simulink model "BBC_ensemble_other"  (R2022a)
settings: Solver=ode15s  StartTime=0.0  StopTime=Tf  RelTol=1e-3  AbsTol=1e-3
PreLoadFcn:
  | Jdamping = 1e-4;
values from neighbouring files (symbols this model uses):
  ball = evalin('base','ball')    [animatedPath.m]
  g = 9.80665    [kinova_params.m]
  max_torque = 0.25    [kinova_params.m]
  plate = evalin('base','plate')    [animatedPath.m]
  R1_q0 = 0    [kinova_params.m]
  R2_q0 = deg2rad(20)    [kinova_params.m]
  R3_q0 = 0    [kinova_params.m]
  R4_q0 = deg2rad(135)    [kinova_params.m]
  R5_q0 = 0    [kinova_params.m]
  U0 = [wrist_torque_0 hand_torque_0]    [kinova_params.m]
undefined symbols (not defined in the file or in its folder): actionTable, actionToIndex, actionUB1, actionUB2, ballWeight, isAvg, isPred, isTerminate, isVote, plateWeight, rewardToIndex, rewardUB1, rewardUB2, stableWeight, stateTable, tranTable, X, Y, Z
libraries: sm_lib x96, nesl_utility x18, rllib x9, dspstat3 x2, simulink x2
(part 3 of 3)

== system BBC_ensemble_other/Kinova Ball Balance/7 DOF Manipulator/Wrist1_Link ==
  Actuator5_AxisInvTransform : sm_lib/Frames and Transforms/Rigid Transform  TranslationMethod=Cartesian  TranslationStandardOffset=0  TranslationLengthUnit=m  TranslationStandardAxis=+Z  TranslationCartesianOffset=[0, 0, 0]  TranslationROffset=0  TranslationROffsetUnits=m  TranslationZOffset=0  TranslationZOffsetUnits=m  TranslationThetaOffset=0  TranslationThetaOffsetUnits=deg  RotationMethod=ArbitraryAxis  RotationAngleUnits=rad  RotationStandardAxis=+Z  RotationAngle=0  RotationArbitraryAxis=[1, 0, 0]  FollAlignAxisA=+X  BaseAlignAxisA=+Y  FollAlignAxisB=+Y  BaseAlignAxisB=+Z  RotationSequenceAxes=FollowerAxes  RotationSequence=XYX  RotationSequenceAngles=[0 0 0]  RotationSequenceAnglesUnits=deg  RotationMatrix=[1 0 0; 0 1 0; 0 0 1]
  Actuator6_AxisTransform : sm_lib/Frames and Transforms/Rigid Transform  TranslationMethod=Cartesian  TranslationStandardOffset=0  TranslationLengthUnit=m  TranslationStandardAxis=+Z  TranslationCartesianOffset=[0, 0, 0]  TranslationROffset=0  TranslationROffsetUnits=m  TranslationZOffset=0  TranslationZOffsetUnits=m  TranslationThetaOffset=0  TranslationThetaOffsetUnits=deg  RotationMethod=ArbitraryAxis  RotationAngleUnits=rad  RotationStandardAxis=+Z  RotationAngle=0  RotationArbitraryAxis=[1, 0, 0]  FollAlignAxisA=+X  BaseAlignAxisA=+Y  FollAlignAxisB=+Y  BaseAlignAxisB=+Z  RotationSequenceAxes=FollowerAxes  RotationSequence=XYX  RotationSequenceAngles=[0 0 0]  RotationSequenceAnglesUnits=deg  RotationMatrix=[1 0 0; 0 1 0; 0 0 1]
  Actuator6_OriginTransform : sm_lib/Frames and Transforms/Rigid Transform  TranslationMethod=Cartesian  TranslationStandardOffset=0  TranslationLengthUnit=m  TranslationStandardAxis=+Z  TranslationCartesianOffset=[0, 0.00017505, -0.10593]  TranslationROffset=0  TranslationROffsetUnits=m  TranslationZOffset=0  TranslationZOffsetUnits=m  TranslationThetaOffset=0  TranslationThetaOffsetUnits=deg  RotationMethod=RotationSequence  RotationAngleUnits=deg  RotationStandardAxis=+Z  RotationAngle=0.0  RotationArbitraryAxis=[0 0 1]  FollAlignAxisA=+X  BaseAlignAxisA=+Y  FollAlignAxisB=+Y  BaseAlignAxisB=+Z  RotationSequenceAxes=BaseAxes  RotationSequence=XYZ  RotationSequenceAngles=[1.5708, 0, 0]  RotationSequenceAnglesUnits=rad  RotationMatrix=[1 0 0; 0 1 0; 0 0 1]
  Inertia : sm_lib/Body Elements/Inertia  InertiaType=Custom  Mass=0.654  MassUnits=kg  CenterOfMass=[0, 0, 0]  CenterOfMassUnits=m  MomentsOfInertia=[0.0013311, 0.0013282, 0.00030696]  MomentsOfInertiaUnits=kg*m^2  ProductsOfInertia=[-0.00022936, -4.267800000000005e-10, -4.584900000000001e-10]  ProductsOfInertiaUnits=kg*m^2  GraphicType=None  MarkerShape=Inertia  MarkerSize=20  GraphicVisPropType=SimpleVisualProperties  GraphicDiffuseColor=[0.5 0.5 0.5]  GraphicSpecularColor=[0.5 0.5 0.5 1.0]  GraphicAmbientColor=[0.15 0.15 0.15 1.0]  GraphicEmissiveColor=[0.0 0.0 0.0 1.0]  GraphicShininess=75  GraphicOpacity=1.0
  InertiaOriginTransform : sm_lib/Frames and Transforms/Rigid Transform  TranslationMethod=Cartesian  TranslationStandardOffset=0  TranslationLengthUnit=m  TranslationStandardAxis=+Z  TranslationCartesianOffset=[-3.2964e-07, -0.009617000000000001, -0.062968]  TranslationROffset=0  TranslationROffsetUnits=m  TranslationZOffset=0  TranslationZOffsetUnits=m  TranslationThetaOffset=0  TranslationThetaOffsetUnits=deg  RotationMethod=RotationSequence  RotationAngleUnits=deg  RotationStandardAxis=+Z  RotationAngle=0.0  RotationArbitraryAxis=[0 0 1]  FollAlignAxisA=+X  BaseAlignAxisA=+Y  FollAlignAxisB=+Y  BaseAlignAxisB=+Z  RotationSequenceAxes=BaseAxes  RotationSequence=XYZ  RotationSequenceAngles=[0, 0, 0]  RotationSequenceAnglesUnits=rad  RotationMatrix=[1 0 0; 0 1 0; 0 0 1]
  ReferenceFrame : sm_lib/Frames and Transforms/Reference Frame
  VisualOriginTransform : sm_lib/Frames and Transforms/Rigid Transform  TranslationMethod=Cartesian  TranslationStandardOffset=0  TranslationLengthUnit=m  TranslationStandardAxis=+Z  TranslationCartesianOffset=[0, 0, 0]  TranslationROffset=0  TranslationROffsetUnits=m  TranslationZOffset=0  TranslationZOffsetUnits=m  TranslationThetaOffset=0  TranslationThetaOffsetUnits=deg  RotationMethod=RotationSequence  RotationAngleUnits=deg  RotationStandardAxis=+Z  RotationAngle=0.0  RotationArbitraryAxis=[0 0 1]  FollAlignAxisA=+X  BaseAlignAxisA=+Y  FollAlignAxisB=+Y  BaseAlignAxisB=+Z  RotationSequenceAxes=BaseAxes  RotationSequence=XYZ  RotationSequenceAngles=[0, 0, 0]  RotationSequenceAnglesUnits=rad  RotationMatrix=[1 0 0; 0 1 0; 0 0 1]
  Wrist1 Link : Subsystem  Variant=on  VariantControlMode=label  VariantControl=Choice  LabelModeActiveChoice=Choice
  F : PMIOPort  Side=Left
  F1 : PMIOPort  Port=2  Side=Right
  connections:
  Actuator5_AxisInvTransform/RConn1 -- F/RConn1
  Actuator6_AxisTransform/RConn1 -- F1/RConn1
  Actuator6_AxisTransform/LConn1 -- Actuator6_OriginTransform/RConn1
  Inertia/RConn1 -- InertiaOriginTransform/RConn1
  Actuator6_OriginTransform/LConn1 -- Actuator5_AxisInvTransform/LConn1 -- InertiaOriginTransform/LConn1 -- VisualOriginTransform/LConn1 -- ReferenceFrame/RConn1
  VisualOriginTransform/RConn1 -- Wrist1 Link/RConn1

== system BBC_ensemble_other/Kinova Ball Balance/7 DOF Manipulator/Wrist2_Link ==
  Actuator6_AxisInvTransform : sm_lib/Frames and Transforms/Rigid Transform  TranslationMethod=Cartesian  TranslationStandardOffset=0  TranslationLengthUnit=m  TranslationStandardAxis=+Z  TranslationCartesianOffset=[0, 0, 0]  TranslationROffset=0  TranslationROffsetUnits=m  TranslationZOffset=0  TranslationZOffsetUnits=m  TranslationThetaOffset=0  TranslationThetaOffsetUnits=deg  RotationMethod=ArbitraryAxis  RotationAngleUnits=rad  RotationStandardAxis=+Z  RotationAngle=0  RotationArbitraryAxis=[1, 0, 0]  FollAlignAxisA=+X  BaseAlignAxisA=+Y  FollAlignAxisB=+Y  BaseAlignAxisB=+Z  RotationSequenceAxes=FollowerAxes  RotationSequence=XYX  RotationSequenceAngles=[0 0 0]  RotationSequenceAnglesUnits=deg  RotationMatrix=[1 0 0; 0 1 0; 0 0 1]
  Actuator7_AxisTransform : sm_lib/Frames and Transforms/Rigid Transform  TranslationMethod=Cartesian  TranslationStandardOffset=0  TranslationLengthUnit=m  TranslationStandardAxis=+Z  TranslationCartesianOffset=[0, 0, 0]  TranslationROffset=0  TranslationROffsetUnits=m  TranslationZOffset=0  TranslationZOffsetUnits=m  TranslationThetaOffset=0  TranslationThetaOffsetUnits=deg  RotationMethod=ArbitraryAxis  RotationAngleUnits=rad  RotationStandardAxis=+Z  RotationAngle=0  RotationArbitraryAxis=[1, 0, 0]  FollAlignAxisA=+X  BaseAlignAxisA=+Y  FollAlignAxisB=+Y  BaseAlignAxisB=+Z  RotationSequenceAxes=FollowerAxes  RotationSequence=XYX  RotationSequenceAngles=[0 0 0]  RotationSequenceAnglesUnits=deg  RotationMatrix=[1 0 0; 0 1 0; 0 0 1]
  Actuator7_OriginTransform : sm_lib/Frames and Transforms/Rigid Transform  TranslationMethod=Cartesian  TranslationStandardOffset=0  TranslationLengthUnit=m  TranslationStandardAxis=+Z  TranslationCartesianOffset=[0, -0.10593, -0.00017505]  TranslationROffset=0  TranslationROffsetUnits=m  TranslationZOffset=0  TranslationZOffsetUnits=m  TranslationThetaOffset=0  TranslationThetaOffsetUnits=deg  RotationMethod=RotationSequence  RotationAngleUnits=deg  RotationStandardAxis=+Z  RotationAngle=0.0  RotationArbitraryAxis=[0 0 1]  FollAlignAxisA=+X  BaseAlignAxisA=+Y  FollAlignAxisB=+Y  BaseAlignAxisB=+Z  RotationSequenceAxes=BaseAxes  RotationSequence=XYZ  RotationSequenceAngles=[-1.5708, 0, 0]  RotationSequenceAnglesUnits=rad  RotationMatrix=[1 0 0; 0 1 0; 0 0 1]
  Inertia : sm_lib/Body Elements/Inertia  InertiaType=Custom  Mass=0.654  MassUnits=kg  CenterOfMass=[0, 0, 0]  CenterOfMassUnits=m  MomentsOfInertia=[0.0013422, 0.00031025, 0.001336]  MomentsOfInertiaUnits=kg*m^2  ProductsOfInertia=[0.00023506, -7.338199999999999e-10, 4.959600000000004e-10]  ProductsOfInertiaUnits=kg*m^2  GraphicType=None  MarkerShape=Inertia  MarkerSize=20  GraphicVisPropType=SimpleVisualProperties  GraphicDiffuseColor=[0.5 0.5 0.5]  GraphicSpecularColor=[0.5 0.5 0.5 1.0]  GraphicAmbientColor=[0.15 0.15 0.15 1.0]  GraphicEmissiveColor=[0.0 0.0 0.0 1.0]  GraphicShininess=75  GraphicOpacity=1.0
  InertiaOriginTransform : sm_lib/Frames and Transforms/Rigid Transform  TranslationMethod=Cartesian  TranslationStandardOffset=0  TranslationLengthUnit=m  TranslationStandardAxis=+Z  TranslationCartesianOffset=[-3.4377e-07, -0.044043, -0.0097804]  TranslationROffset=0  TranslationROffsetUnits=m  TranslationZOffset=0  TranslationZOffsetUnits=m  TranslationThetaOffset=0  TranslationThetaOffsetUnits=deg  RotationMethod=RotationSequence  RotationAngleUnits=deg  RotationStandardAxis=+Z  RotationAngle=0.0  RotationArbitraryAxis=[0 0 1]  FollAlignAxisA=+X  BaseAlignAxisA=+Y  FollAlignAxisB=+Y  BaseAlignAxisB=+Z  RotationSequenceAxes=BaseAxes  RotationSequence=XYZ  RotationSequenceAngles=[0, 0, 0]  RotationSequenceAnglesUnits=rad  RotationMatrix=[1 0 0; 0 1 0; 0 0 1]
  ReferenceFrame : sm_lib/Frames and Transforms/Reference Frame
  VisualOriginTransform : sm_lib/Frames and Transforms/Rigid Transform  TranslationMethod=Cartesian  TranslationStandardOffset=0  TranslationLengthUnit=m  TranslationStandardAxis=+Z  TranslationCartesianOffset=[0, 0, 0]  TranslationROffset=0  TranslationROffsetUnits=m  TranslationZOffset=0  TranslationZOffsetUnits=m  TranslationThetaOffset=0  TranslationThetaOffsetUnits=deg  RotationMethod=RotationSequence  RotationAngleUnits=deg  RotationStandardAxis=+Z  RotationAngle=0.0  RotationArbitraryAxis=[0 0 1]  FollAlignAxisA=+X  BaseAlignAxisA=+Y  FollAlignAxisB=+Y  BaseAlignAxisB=+Z  RotationSequenceAxes=BaseAxes  RotationSequence=XYZ  RotationSequenceAngles=[0, 0, 0]  RotationSequenceAnglesUnits=rad  RotationMatrix=[1 0 0; 0 1 0; 0 0 1]
  Wrist2 Link : Subsystem  Variant=on  VariantControlMode=label  VariantControl=Choice  LabelModeActiveChoice=Choice
  F : PMIOPort  Side=Left
  F1 : PMIOPort  Port=2  Side=Right
  connections:
  Actuator6_AxisInvTransform/RConn1 -- F/RConn1
  Actuator7_AxisTransform/RConn1 -- F1/RConn1
  Actuator7_AxisTransform/LConn1 -- Actuator7_OriginTransform/RConn1
  Inertia/RConn1 -- InertiaOriginTransform/RConn1
  Actuator7_OriginTransform/LConn1 -- Actuator6_AxisInvTransform/LConn1 -- InertiaOriginTransform/LConn1 -- VisualOriginTransform/LConn1 -- ReferenceFrame/RConn1
  VisualOriginTransform/RConn1 -- Wrist2 Link/RConn1

== system BBC_ensemble_other/Kinova Ball Balance/7 DOF Manipulator/base_link ==
  Actuator1_AxisTransform : sm_lib/Frames and Transforms/Rigid Transform  TranslationMethod=Cartesian  TranslationStandardOffset=0  TranslationLengthUnit=m  TranslationStandardAxis=+Z  TranslationCartesianOffset=[0, 0, 0]  TranslationROffset=0  TranslationROffsetUnits=m  TranslationZOffset=0  TranslationZOffsetUnits=m  TranslationThetaOffset=0  TranslationThetaOffsetUnits=deg  RotationMethod=ArbitraryAxis  RotationAngleUnits=rad  RotationStandardAxis=+Z  RotationAngle=0  RotationArbitraryAxis=[1, 0, 0]  FollAlignAxisA=+X  BaseAlignAxisA=+Y  FollAlignAxisB=+Y  BaseAlignAxisB=+Z  RotationSequenceAxes=FollowerAxes  RotationSequence=XYX  RotationSequenceAngles=[0 0 0]  RotationSequenceAnglesUnits=deg  RotationMatrix=[1 0 0; 0 1 0; 0 0 1]
  Actuator1_OriginTransform : sm_lib/Frames and Transforms/Rigid Transform  TranslationMethod=Cartesian  TranslationStandardOffset=0  TranslationLengthUnit=m  TranslationStandardAxis=+Z  TranslationCartesianOffset=[0, 0, 0.15643]  TranslationROffset=0  TranslationROffsetUnits=m  TranslationZOffset=0  TranslationZOffsetUnits=m  TranslationThetaOffset=0  TranslationThetaOffsetUnits=deg  RotationMethod=RotationSequence  RotationAngleUnits=deg  RotationStandardAxis=+Z  RotationAngle=0.0  RotationArbitraryAxis=[0 0 1]  FollAlignAxisA=+X  BaseAlignAxisA=+Y  FollAlignAxisB=+Y  BaseAlignAxisB=+Z  RotationSequenceAxes=BaseAxes  RotationSequence=XYZ  RotationSequenceAngles=[-3.141585307179587, 0, 0]  RotationSequenceAnglesUnits=rad  RotationMatrix=[1 0 0; 0 1 0; 0 0 1]
  Base Link : Subsystem  Variant=on  VariantControlMode=label  VariantControl=Choice  LabelModeActiveChoice=Choice
  ReferenceFrame : sm_lib/Frames and Transforms/Reference Frame
  F : PMIOPort  Side=Left
  F1 : PMIOPort  Port=2  Side=Right
  connections:
  Actuator1_AxisTransform/RConn1 -- F1/RConn1
  Actuator1_AxisTransform/LConn1 -- Actuator1_OriginTransform/RConn1
  F/RConn1 -- Actuator1_OriginTransform/LConn1 -- ReferenceFrame/RConn1 -- Base Link/RConn1

== system BBC_ensemble_other/Kinova Ball Balance/7 DOF Manipulator/mount ==
  Cylindrical Solid : sm_lib/Body Elements/Cylindrical Solid  GraphicAmbientColor=[0.15 0.15 0.15 1.0]  BasedOnType=Density  CenterOfMass=[0 0 0]  CenterOfMassUnits=m  GraphicDiffuseColor=[0.6 0.6 0.6]  CylinderLength=0.01  CylinderLengthUnits=m  CylinderRadius=0.1  CylinderRadiusUnits=m  Density=1000  DensityUnits=kg/m^3  DoExposeReferenceFrame=off  GraphicEmissiveColor=[0.0 0.0 0.0 1.0]  ExportEntireGeometry=off  SerializedFrames=<Frames><Frame><Id>Frame1</Id><Value><Name>F1</Name><Origin><Source>GeometricFeature</Source><FeatureName>top surface</FeatureName></Origin><PrimaryAxis><DefinedDirection>+Z</DefinedDirection><Source>ReferenceFrame</Source><SourceDirection>+Z</SourceDirection><FeatureName></FeatureName></PrimaryAxis><SecondaryAxis><DefinedDirection>+X</DefinedDirection><Source>ReferenceFrame</Source><SourceDirection>+X</SourceDirection><FeatureName></FeatureName></SecondaryAxis></Value></Frame><Frame><Id>Frame2</Id><Value><Name>F2</Name><Origin><Source>GeometricFeature</Source><FeatureName>bottom surface</FeatureName></Origin><PrimaryAxis><DefinedDirection>+Z</DefinedDirection><Source>ReferenceFrame</Source><SourceDirection>+Z</SourceDirection><FeatureName></FeatureName></PrimaryAxis><SecondaryAxis><DefinedDirection>+X</DefinedDirection><Source>ReferenceFrame</Source><SourceDirection>+X</SourceDirection><FeatureName></FeatureName></SecondaryAxis></Value></Frame></Frames>  MarkerShape=Sphere  MarkerSize=10  GraphicType=FromGeometry  InertiaType=CalculateFromGeometry  Mass=1  MassUnits=kg  MomentsOfInertia=[1 1 1]  MomentsOfInertiaUnits=kg*m^2  GraphicOpacity=1.0  ProductsOfInertia=[0 0 0]  ProductsOfInertiaUnits=kg*m^2  GraphicShininess=75  GraphicSpecularColor=[0.5 0.5 0.5 1.0]  GraphicVisPropType=SimpleVisualProperties
  F : PMIOPort  Side=Right
  F1 : PMIOPort  Port=2  Side=Left
  connections:
  Cylindrical Solid/LConn1 -- F1/RConn1
  F/RConn1 -- Cylindrical Solid/RConn1

== system BBC_ensemble_other/Kinova Ball Balance/7 DOF Manipulator/Bracelet_Link/Bracelet Link ==
  FileSolid : Subsystem  VariantControl=Choice_1
  Inertia : Subsystem  VariantControl=Choice
  R : PMIOPort  Side=Right

== system BBC_ensemble_other/Kinova Ball Balance/7 DOF Manipulator/ForeArm_Link/ForeArm Link ==
  FileSolid : Subsystem  VariantControl=Choice_1
  Inertia : Subsystem  VariantControl=Choice
  R : PMIOPort  Side=Right

== system BBC_ensemble_other/Kinova Ball Balance/7 DOF Manipulator/HalfArm1_Link/HalfArm1 Link ==
  FileSolid : Subsystem  VariantControl=Choice_1
  Inertia : Subsystem  VariantControl=Choice
  R : PMIOPort  Side=Right

== system BBC_ensemble_other/Kinova Ball Balance/7 DOF Manipulator/HalfArm2_Link/HalfArm2 Link ==
  FileSolid : Subsystem  VariantControl=Choice_1
  Inertia : Subsystem  VariantControl=Choice
  R : PMIOPort  Side=Right

== system BBC_ensemble_other/Kinova Ball Balance/7 DOF Manipulator/Shoulder_Link/Shoulder Link ==
  FileSolid : Subsystem  VariantControl=Choice_1
  Inertia : Subsystem  VariantControl=Choice
  R : PMIOPort  Side=Right

== system BBC_ensemble_other/Kinova Ball Balance/7 DOF Manipulator/Wrist1_Link/Wrist1 Link ==
  FileSolid : Subsystem  VariantControl=Choice_1
  Inertia : Subsystem  VariantControl=Choice
  R : PMIOPort  Side=Right

== system BBC_ensemble_other/Kinova Ball Balance/7 DOF Manipulator/Wrist2_Link/Wrist2 Link ==
  FileSolid : Subsystem  VariantControl=Choice_1
  Inertia : Subsystem  VariantControl=Choice
  R : PMIOPort  Side=Right

== system BBC_ensemble_other/Kinova Ball Balance/7 DOF Manipulator/base_link/Base Link ==
  FileSolid : Subsystem  VariantControl=Choice_1
  Inertia : Subsystem  VariantControl=Choice
  R : PMIOPort  Side=Right

== system BBC_ensemble_other/Kinova Ball Balance/7 DOF Manipulator/Bracelet_Link/Bracelet Link/FileSolid ==
  Bracelet Link : sm_lib/Body Elements/File Solid  ExtGeomFileName=bracelet_with_vision_link.STL  UnitType=Custom  ExtGeomFileUnits=m  StepReaderType=HEX  ExportConvexHullGeometry=off  InertiaType=Custom  Mass=0.0639903  MassUnits=kg  CenterOfMass=[-0.000374733, 0.0200972, 0.0397002]  CenterOfMassUnits=m  MomentsOfInertia=[8.77763e-05, 5.386e-05, 0.000111032]  MomentsOfInertiaUnits=kg*m^2  ProductsOfInertia=[-7.81917e-06, 1.77829e-07, -4.01652e-07]  ProductsOfInertiaUnits=kg*m^2  BasedOnType=DensityFromFile  Density=1000  DensityUnits=kg/m^3  DoExposeReferenceFrame=on  SerializedFrames=<Frames/>  GraphicType=FromGeometry  MarkerShape=Sphere  MarkerSize=10  GraphicVisPropType=SimpleVisualProperties  GraphicDiffuseColor=[0.6666667 0.77254903 0.92941177]  GraphicSpecularColor=[0.5 0.5 0.5 1.0]  GraphicAmbientColor=[0.15 0.15 0.15 1.0]  GraphicEmissiveColor=[0.0 0.0 0.0 1.0]  GraphicShininess=75  GraphicOpacity=1
  R : PMIOPort  Side=Right
  connections:
  Bracelet Link/RConn1 -- R/RConn1

== system BBC_ensemble_other/Kinova Ball Balance/7 DOF Manipulator/Bracelet_Link/Bracelet Link/Inertia ==
  Inertia1 : sm_lib/Body Elements/Inertia  InertiaType=Custom  Mass=0.0639903  MassUnits=kg  CenterOfMass=[-0.000374733, 0.0200972, 0.0397002]  CenterOfMassUnits=m  MomentsOfInertia=[8.77763e-05, 5.386e-05, 0.000111032]  MomentsOfInertiaUnits=kg*m^2  ProductsOfInertia=[-7.81917e-06, 1.77829e-07, -4.01652e-07]  ProductsOfInertiaUnits=kg*m^2  GraphicType=Marker  MarkerShape=Inertia  MarkerSize=20  GraphicVisPropType=SimpleVisualProperties  GraphicDiffuseColor=[0.5 0.5 0.5]  GraphicSpecularColor=[0.5 0.5 0.5 1.0]  GraphicAmbientColor=[0.15 0.15 0.15 1.0]  GraphicEmissiveColor=[0.0 0.0 0.0 1.0]  GraphicShininess=75  GraphicOpacity=1.0
  R : PMIOPort  Side=Right
  connections:
  Inertia1/RConn1 -- R/RConn1

== system BBC_ensemble_other/Kinova Ball Balance/7 DOF Manipulator/ForeArm_Link/ForeArm Link/FileSolid ==
  Forearm Link : sm_lib/Body Elements/File Solid  ExtGeomFileName=forearm_link.STL  UnitType=Custom  ExtGeomFileUnits=m  StepReaderType=HEX  ExportConvexHullGeometry=off  InertiaType=Custom  Mass=0.108759  MassUnits=kg  CenterOfMass=[0.0794976, 0.0148416, -8.39544e-07]  CenterOfMassUnits=m  MomentsOfInertia=[0.000118324, 0.000832188, 0.000809477]  MomentsOfInertiaUnits=kg*m^2  ProductsOfInertia=[3.60538e-09, -2.24072e-09, 7.50733e-05]  ProductsOfInertiaUnits=kg*m^2  BasedOnType=DensityFromFile  Density=1000  DensityUnits=kg/m^3  DoExposeReferenceFrame=on  SerializedFrames=<Frames/>  GraphicType=FromGeometry  MarkerShape=Sphere  MarkerSize=10  GraphicVisPropType=SimpleVisualProperties  GraphicDiffuseColor=[0.54509807 0.654902 0.77254903]  GraphicSpecularColor=[0.5 0.5 0.5 1.0]  GraphicAmbientColor=[0.15 0.15 0.15 1.0]  GraphicEmissiveColor=[0.0 0.0 0.0 1.0]  GraphicShininess=75  GraphicOpacity=1
  R : PMIOPort  Side=Right
  connections:
  Forearm Link/RConn1 -- R/RConn1

== system BBC_ensemble_other/Kinova Ball Balance/7 DOF Manipulator/ForeArm_Link/ForeArm Link/Inertia ==
  Inertia1 : sm_lib/Body Elements/Inertia  InertiaType=Custom  Mass=0.108759  MassUnits=kg  CenterOfMass=[0.0794976, 0.0148416, -8.39544e-07]  CenterOfMassUnits=m  MomentsOfInertia=[0.000118324, 0.000832188, 0.000809477]  MomentsOfInertiaUnits=kg*m^2  ProductsOfInertia=[3.60538e-09, -2.24072e-09, 7.50733e-05]  ProductsOfInertiaUnits=kg*m^2  GraphicType=Marker  MarkerShape=Inertia  MarkerSize=20  GraphicVisPropType=SimpleVisualProperties  GraphicDiffuseColor=[0.5 0.5 0.5]  GraphicSpecularColor=[0.5 0.5 0.5 1.0]  GraphicAmbientColor=[0.15 0.15 0.15 1.0]  GraphicEmissiveColor=[0.0 0.0 0.0 1.0]  GraphicShininess=75  GraphicOpacity=1.0
  R : PMIOPort  Side=Right
  connections:
  Inertia1/RConn1 -- R/RConn1

== system BBC_ensemble_other/Kinova Ball Balance/7 DOF Manipulator/HalfArm1_Link/HalfArm1 Link/FileSolid ==
  Half Arm1 Link : sm_lib/Body Elements/File Solid  ExtGeomFileName=half_arm_1_link.STL  UnitType=Custom  ExtGeomFileUnits=m  StepReaderType=HEX  ExportConvexHullGeometry=off  InertiaType=Custom  Mass=0.137977  MassUnits=kg  CenterOfMass=[0.100808, 0.0121234, 4.10274e-06]  CenterOfMassUnits=m  MomentsOfInertia=[0.000202425, 0.00113112, 0.00110619]  MomentsOfInertiaUnits=kg*m^2  ProductsOfInertia=[1.72409e-08, -8.98835e-09, 0.000105223]  ProductsOfInertiaUnits=kg*m^2  BasedOnType=DensityFromFile  Density=1000  DensityUnits=kg/m^3  DoExposeReferenceFrame=on  SerializedFrames=<Frames/>  GraphicType=FromGeometry  MarkerShape=Sphere  MarkerSize=10  GraphicVisPropType=SimpleVisualProperties  GraphicDiffuseColor=[0.54509807 0.654902 0.77254903]  GraphicSpecularColor=[0.5 0.5 0.5 1.0]  GraphicAmbientColor=[0.15 0.15 0.15 1.0]  GraphicEmissiveColor=[0.0 0.0 0.0 1.0]  GraphicShininess=75  GraphicOpacity=1
  R : PMIOPort  Side=Right
  connections:
  Half Arm1 Link/RConn1 -- R/RConn1

== system BBC_ensemble_other/Kinova Ball Balance/7 DOF Manipulator/HalfArm1_Link/HalfArm1 Link/Inertia ==
  Inertia1 : sm_lib/Body Elements/Inertia  InertiaType=Custom  Mass=0.137977  MassUnits=kg  CenterOfMass=[0.100808, 0.0121234, 4.10274e-06]  CenterOfMassUnits=m  MomentsOfInertia=[0.000202425, 0.00113112, 0.00110619]  MomentsOfInertiaUnits=kg*m^2  ProductsOfInertia=[1.72409e-08, -8.98835e-09, 0.000105223]  ProductsOfInertiaUnits=kg*m^2  GraphicType=Marker  MarkerShape=Inertia  MarkerSize=20  GraphicVisPropType=SimpleVisualProperties  GraphicDiffuseColor=[0.5 0.5 0.5]  GraphicSpecularColor=[0.5 0.5 0.5 1.0]  GraphicAmbientColor=[0.15 0.15 0.15 1.0]  GraphicEmissiveColor=[0.0 0.0 0.0 1.0]  GraphicShininess=75  GraphicOpacity=1.0
  R : PMIOPort  Side=Right
  connections:
  Inertia1/RConn1 -- R/RConn1

== system BBC_ensemble_other/Kinova Ball Balance/7 DOF Manipulator/HalfArm2_Link/HalfArm2 Link/FileSolid ==
  Half Arm2 Link : sm_lib/Body Elements/File Solid  ExtGeomFileName=half_arm_2_link.STL  UnitType=Custom  ExtGeomFileUnits=m  StepReaderType=HEX  ExportConvexHullGeometry=off  InertiaType=Custom  Mass=0.137978  MassUnits=kg  CenterOfMass=[0.0871838, 0.0118108, 4.16659e-06]  CenterOfMassUnits=m  MomentsOfInertia=[0.000195075, 0.0011006, 0.00106833]  MomentsOfInertiaUnits=kg*m^2  ProductsOfInertia=[1.66656e-08, -1.69023e-08, 7.86653e-05]  ProductsOfInertiaUnits=kg*m^2  BasedOnType=DensityFromFile  Density=1000  DensityUnits=kg/m^3  DoExposeReferenceFrame=on  SerializedFrames=<Frames/>  GraphicType=FromGeometry  MarkerShape=Sphere  MarkerSize=10  GraphicVisPropType=SimpleVisualProperties  GraphicDiffuseColor=[0.6666667 0.77254903 0.92941177]  GraphicSpecularColor=[0.5 0.5 0.5 1.0]  GraphicAmbientColor=[0.15 0.15 0.15 1.0]  GraphicEmissiveColor=[0.0 0.0 0.0 1.0]  GraphicShininess=75  GraphicOpacity=1
  R : PMIOPort  Side=Right
  connections:
  Half Arm2 Link/RConn1 -- R/RConn1

== system BBC_ensemble_other/Kinova Ball Balance/7 DOF Manipulator/HalfArm2_Link/HalfArm2 Link/Inertia ==
  Inertia1 : sm_lib/Body Elements/Inertia  InertiaType=Custom  Mass=0.137978  MassUnits=kg  CenterOfMass=[0.0871838, 0.0118108, 4.16659e-06]  CenterOfMassUnits=m  MomentsOfInertia=[0.000195075, 0.0011006, 0.00106833]  MomentsOfInertiaUnits=kg*m^2  ProductsOfInertia=[1.66656e-08, -1.69023e-08, 7.86653e-05]  ProductsOfInertiaUnits=kg*m^2  GraphicType=Marker  MarkerShape=Inertia  MarkerSize=20  GraphicVisPropType=SimpleVisualProperties  GraphicDiffuseColor=[0.5 0.5 0.5]  GraphicSpecularColor=[0.5 0.5 0.5 1.0]  GraphicAmbientColor=[0.15 0.15 0.15 1.0]  GraphicEmissiveColor=[0.0 0.0 0.0 1.0]  GraphicShininess=75  GraphicOpacity=1.0
  R : PMIOPort  Side=Right
  connections:
  Inertia1/RConn1 -- R/RConn1

== system BBC_ensemble_other/Kinova Ball Balance/7 DOF Manipulator/Shoulder_Link/Shoulder Link/FileSolid ==
  Shoulder Link : sm_lib/Body Elements/File Solid  ExtGeomFileName=shoulder_link.STL  UnitType=Custom  ExtGeomFileUnits=m  StepReaderType=HEX  ExportConvexHullGeometry=off  InertiaType=Custom  Mass=0.206679  MassUnits=kg  CenterOfMass=[0.0758362, 0.0170163, 7.48345e-07]  CenterOfMassUnits=m  MomentsOfInertia=[0.000301623, 0.000658228, 0.000584422]  MomentsOfInertiaUnits=kg*m^2  ProductsOfInertia=[6.12368e-09, 4.93274e-09, -6.36892e-05]  ProductsOfInertiaUnits=kg*m^2  BasedOnType=DensityFromFile  Density=1000  DensityUnits=kg/m^3  DoExposeReferenceFrame=on  SerializedFrames=<Frames/>  GraphicType=FromGeometry  MarkerShape=Sphere  MarkerSize=10  GraphicVisPropType=SimpleVisualProperties  GraphicDiffuseColor=[0.6666667 0.77254903 0.92941177]  GraphicSpecularColor=[0.5 0.5 0.5 1.0]  GraphicAmbientColor=[0.15 0.15 0.15 1.0]  GraphicEmissiveColor=[0.0 0.0 0.0 1.0]  GraphicShininess=75  GraphicOpacity=1
  R : PMIOPort  Side=Right
  connections:
  R/RConn1 -- Shoulder Link/RConn1

== system BBC_ensemble_other/Kinova Ball Balance/7 DOF Manipulator/Shoulder_Link/Shoulder Link/Inertia ==
  Inertia1 : sm_lib/Body Elements/Inertia  InertiaType=Custom  Mass=0.206679  MassUnits=kg  CenterOfMass=[0.0758362, 0.0170163, 7.48345e-07]  CenterOfMassUnits=m  MomentsOfInertia=[0.000301623, 0.000658228, 0.000584422]  MomentsOfInertiaUnits=kg*m^2  ProductsOfInertia=[6.12368e-09, 4.93274e-09, -6.36892e-05]  ProductsOfInertiaUnits=kg*m^2  GraphicType=Marker  MarkerShape=Inertia  MarkerSize=20  GraphicVisPropType=SimpleVisualProperties  GraphicDiffuseColor=[0.5 0.5 0.5]  GraphicSpecularColor=[0.5 0.5 0.5 1.0]  GraphicAmbientColor=[0.15 0.15 0.15 1.0]  GraphicEmissiveColor=[0.0 0.0 0.0 1.0]  GraphicShininess=75  GraphicOpacity=1.0
  R : PMIOPort  Side=Right
  connections:
  Inertia1/RConn1 -- R/RConn1

== system BBC_ensemble_other/Kinova Ball Balance/7 DOF Manipulator/Wrist1_Link/Wrist1 Link/FileSolid ==
  Wrist1 Link : sm_lib/Body Elements/File Solid  ExtGeomFileName=spherical_wrist_1_link.STL  UnitType=Custom  ExtGeomFileUnits=m  StepReaderType=HEX  ExportConvexHullGeometry=off  InertiaType=Custom  Mass=0.0607261  MassUnits=kg  CenterOfMass=[0.0669267, 0.0134734, -3.64177e-07]  CenterOfMassUnits=m  MomentsOfInertia=[5.88928e-05, 0.000140521, 0.000138155]  MomentsOfInertiaUnits=kg*m^2  ProductsOfInertia=[2.83121e-09, 1.56006e-09, -2.20674e-05]  ProductsOfInertiaUnits=kg*m^2  BasedOnType=DensityFromFile  Density=1000  DensityUnits=kg/m^3  DoExposeReferenceFrame=on  SerializedFrames=<Frames/>  GraphicType=FromGeometry  MarkerShape=Sphere  MarkerSize=10  GraphicVisPropType=SimpleVisualProperties  GraphicDiffuseColor=[0.6666667 0.77254903 0.92941177]  GraphicSpecularColor=[0.5 0.5 0.5 1.0]  GraphicAmbientColor=[0.15 0.15 0.15 1.0]  GraphicEmissiveColor=[0.0 0.0 0.0 1.0]  GraphicShininess=75  GraphicOpacity=1
  R : PMIOPort  Side=Right
  connections:
  Wrist1 Link/RConn1 -- R/RConn1

== system BBC_ensemble_other/Kinova Ball Balance/7 DOF Manipulator/Wrist1_Link/Wrist1 Link/Inertia ==
  Inertia1 : sm_lib/Body Elements/Inertia  InertiaType=Custom  Mass=0.0607261  MassUnits=kg  CenterOfMass=[0.0669267, 0.0134734, -3.64177e-07]  CenterOfMassUnits=m  MomentsOfInertia=[5.88928e-05, 0.000140521, 0.000138155]  MomentsOfInertiaUnits=kg*m^2  ProductsOfInertia=[2.83121e-09, 1.56006e-09, -2.20674e-05]  ProductsOfInertiaUnits=kg*m^2  GraphicType=Marker  MarkerShape=Inertia  MarkerSize=20  GraphicVisPropType=SimpleVisualProperties  GraphicDiffuseColor=[0.5 0.5 0.5]  GraphicSpecularColor=[0.5 0.5 0.5 1.0]  GraphicAmbientColor=[0.15 0.15 0.15 1.0]  GraphicEmissiveColor=[0.0 0.0 0.0 1.0]  GraphicShininess=75  GraphicOpacity=1.0
  R : PMIOPort  Side=Right
  connections:
  Inertia1/RConn1 -- R/RConn1

== system BBC_ensemble_other/Kinova Ball Balance/7 DOF Manipulator/Wrist2_Link/Wrist2 Link/FileSolid ==
  Wrist2 Link : sm_lib/Body Elements/File Solid  ExtGeomFileName=spherical_wrist_2_link.STL  UnitType=Custom  ExtGeomFileUnits=m  StepReaderType=HEX  ExportConvexHullGeometry=off  InertiaType=Custom  Mass=0.0607235  MassUnits=kg  CenterOfMass=[0.0566892, 0.0133552, 2.07599e-07]  CenterOfMassUnits=m  MomentsOfInertia=[6.22269e-05, 0.000150545, 0.000151516]  MomentsOfInertiaUnits=kg*m^2  ProductsOfInertia=[-8.5602e-09, -1.23542e-08, -3.01223e-05]  ProductsOfInertiaUnits=kg*m^2  BasedOnType=DensityFromFile  Density=1000  DensityUnits=kg/m^3  DoExposeReferenceFrame=on  SerializedFrames=<Frames/>  GraphicType=FromGeometry  MarkerShape=Sphere  MarkerSize=10  GraphicVisPropType=SimpleVisualProperties  GraphicDiffuseColor=[0.54509807 0.654902 0.77254903]  GraphicSpecularColor=[0.5 0.5 0.5 1.0]  GraphicAmbientColor=[0.15 0.15 0.15 1.0]  GraphicEmissiveColor=[0.0 0.0 0.0 1.0]  GraphicShininess=75  GraphicOpacity=1
  R : PMIOPort  Side=Right
  connections:
  Wrist2 Link/RConn1 -- R/RConn1

== system BBC_ensemble_other/Kinova Ball Balance/7 DOF Manipulator/Wrist2_Link/Wrist2 Link/Inertia ==
  Inertia1 : sm_lib/Body Elements/Inertia  InertiaType=Custom  Mass=0.0607235  MassUnits=kg  CenterOfMass=[0.0566892, 0.0133552, 2.07599e-07]  CenterOfMassUnits=m  MomentsOfInertia=[6.22269e-05, 0.000150545, 0.000151516]  MomentsOfInertiaUnits=kg*m^2  ProductsOfInertia=[-8.5602e-09, -1.23542e-08, -3.01223e-05]  ProductsOfInertiaUnits=kg*m^2  GraphicType=Marker  MarkerShape=Inertia  MarkerSize=20  GraphicVisPropType=SimpleVisualProperties  GraphicDiffuseColor=[0.5 0.5 0.5]  GraphicSpecularColor=[0.5 0.5 0.5 1.0]  GraphicAmbientColor=[0.15 0.15 0.15 1.0]  GraphicEmissiveColor=[0.0 0.0 0.0 1.0]  GraphicShininess=75  GraphicOpacity=1.0
  R : PMIOPort  Side=Right
  connections:
  Inertia1/RConn1 -- R/RConn1

== system BBC_ensemble_other/Kinova Ball Balance/7 DOF Manipulator/base_link/Base Link/FileSolid ==
  Base Link : sm_lib/Body Elements/File Solid  ExtGeomFileName=base_link.STL  UnitType=Custom  ExtGeomFileUnits=m  StepReaderType=HEX  ExportConvexHullGeometry=off  InertiaType=Custom  Mass=1.06185  MassUnits=kg  CenterOfMass=[0.000712614, 0.0763467, 0.000106583]  CenterOfMassUnits=m  MomentsOfInertia=[0.00275492, 0.0011525, 0.00277912]  MomentsOfInertiaUnits=kg*m^2  ProductsOfInertia=[-1.84082e-06, 1.0557e-07, 2.81404e-05]  ProductsOfInertiaUnits=kg*m^2  BasedOnType=DensityFromFile  Density=1000  DensityUnits=kg/m^3  DoExposeReferenceFrame=on  SerializedFrames=<Frames/>  GraphicType=FromGeometry  MarkerShape=Sphere  MarkerSize=10  GraphicVisPropType=SimpleVisualProperties  GraphicDiffuseColor=[0.54509807 0.654902 0.77254903]  GraphicSpecularColor=[0.5 0.5 0.5 1.0]  GraphicAmbientColor=[0.15 0.15 0.15 1.0]  GraphicEmissiveColor=[0.0 0.0 0.0 1.0]  GraphicShininess=75  GraphicOpacity=1
  R : PMIOPort  Side=Right
  connections:
  Base Link/RConn1 -- R/RConn1

== system BBC_ensemble_other/Kinova Ball Balance/7 DOF Manipulator/base_link/Base Link/Inertia ==
  Inertia : sm_lib/Body Elements/Inertia  InertiaType=Custom  Mass=1.06185  MassUnits=kg  CenterOfMass=[0.000712614, 0.0763467, 0.000106583]  CenterOfMassUnits=m  MomentsOfInertia=[0.00275492, 0.0011525, 0.00277912]  MomentsOfInertiaUnits=kg*m^2  ProductsOfInertia=[-1.84082e-06, 1.0557e-07, 2.81404e-05]  ProductsOfInertiaUnits=kg*m^2  GraphicType=Marker  MarkerShape=Inertia  MarkerSize=20  GraphicVisPropType=SimpleVisualProperties  GraphicDiffuseColor=[0.5 0.5 0.5]  GraphicSpecularColor=[0.5 0.5 0.5 1.0]  GraphicAmbientColor=[0.15 0.15 0.15 1.0]  GraphicEmissiveColor=[0.0 0.0 0.0 1.0]  GraphicShininess=75  GraphicOpacity=1.0
  R : PMIOPort  Side=Right
  connections:
  Inertia/RConn1 -- R/RConn1

== matlab function BBC_ensemble_other/Kinova Ball Balance/Reward/Quaternions to Rotation Angles ZYX sequence ==
  data: q input; tilt output
function tilt = quat2tilt(q)
% Quaternion to Euler angle transformation
% Source: https://en.wikipedia.org/wiki/Conversion_between_quaternions_and_Euler_angles

% unpack quaternion
q0 = q(1);
q1 = q(2);
q2 = q(3);
q3 = q(4);

tilt = zeros(3,1);

% tilt about X axis (tilt_y or roll)
tilt(3) = atan2(2*(q0*q1+q2*q3),1-2*(q1^2+q2^2));

% tilt about Y axis (tilt_x or pitch)
tilt(2) = asin(2*(q0*q2-q3*q1));

% tilt about Z axis (yaw)
tilt(1) = atan2(2*(q0*q3+q2*q1),1-2*(q2^2+q3^2));

== matlab function BBC_ensemble_other/Ensemble Control System/Semantics Prediction/MATLAB Function ==
  data: actionJ6 input; actionJ7 input; nextReward output; reward input; actionUB_1 input; actionUB_2 input; actionToIndexTable input; rewardUB_1 input; rewardUB_2 input; rewardToIndexTable input; tranTable input; stateTable input; actionTable input
function nextReward  = fcn(actionJ6,actionJ7,reward, actionUB_1,actionUB_2,actionToIndexTable,rewardUB_1,rewardUB_2, rewardToIndexTable, tranTable, stateTable,actionTable)

numController = 9;

nextReward = ones(numController, 1);
abReward_1 = find(rewardUB_1 >= reward(1), 1, 'first');  % concrete state -> abstract state
abReward_2 = find(rewardUB_2 >= reward(2), 1, 'first');

if isempty(abReward_1) || isempty(abReward_2)      % if this is an unseen reward
    nextReward = zeros(numController,1);
else
    rewardIndex1 = rewardToIndexTable(:,1)==abReward_1;
    rewardIndex2 = rewardToIndexTable(:,2)==abReward_2;
    
    if isempty(rewardIndex1) || isempty(rewardIndex2)      % if this is an unseen abstract state
        nextReward = zeros(numController,1);
    else
        abState = rewardToIndexTable(rewardIndex1 & rewardIndex2, 3);
        
        if isempty(abState)
            nextReward = zeros(numController,1);
        else
            for i = 1:numController
                
                action_1 = actionJ6(i);
                action_2 = actionJ7(i);
                abAction_1 = find(actionUB_1 >= action_1, 1, 'first'); % concrete action -> abstract action
                abAction_2 = find(actionUB_2 >= action_2, 1, 'first');

                actionIndex1 = actionToIndexTable(:,1)==abAction_1;
                actionIndex2 = actionToIndexTable(:,2)==abAction_2;

                if isempty(actionIndex1) || isempty(actionIndex2)
                    % nextReward = zeros(numController,1);
                    nextReward(i,1) = 0;
                    % break;
                else
                    abAction = actionToIndexTable(actionToIndexTable(:,1)==abAction_1 & actionToIndexTable(:,2)==abAction_2,3);

                    if isempty(abAction)
                        % nextReward = zeros(numController,1);
                        nextReward(i,1) = 0;
                        % break;
                    else
                        stateIndex = stateTable==abState;
                        actionindex = actionTable==abAction;

                        if isempty(stateIndex) || isempty(actionindex)  % if this is an unseen abstract state-action pair
                            abTranReward = 0;
                        else
                            temp = stateIndex + actionindex;
                            if ismember(2,temp)
                                abTranReward = tranTable((stateIndex & actionindex),5);
                            else
                                abTranReward = 0;
                            end
                        end
                        nextReward(i,1) = abTranReward;
                    end
                end
            end
        end
    end
end

== matlab function BBC_ensemble_other/Ensemble Control System/vote and average/majority voting ==
  data: actionOut output; actionJ6 input; actionJ7 input; actionUB_1 input; actionUB_2 input
function actionOut = fcn(actionJ6, actionJ7, actionUB_1,actionUB_2)

numController = 9;

abstractActionJ6 = zeros(numController, 2);
abstractActionJ7 = zeros(numController, 2);


for i = 1:numController
    abstractActionJ6(i,1) = find(actionUB_1 >= actionJ6(i), 1, 'first');      % concrete action -> abstract action;
    abstractActionJ6(i,2) = actionJ6(i);
    abstractActionJ7(i,1) = find(actionUB_2 >= actionJ7(i), 1, 'first');      % concrete action -> abstract action;
    abstractActionJ7(i,2) = actionJ7(i);
end

[GC,GR] = groupcounts(abstractActionJ6(:,1));
actionIndexJ6 = GR(GC==max(GC));
actionIndexJ6 = ismember(abstractActionJ6(:,1),actionIndexJ6);

[GC,GR] = groupcounts(abstractActionJ7(:,1));
actionIndexJ7 = GR(GC==max(GC));
actionIndexJ7 = ismember(abstractActionJ7(:,1),actionIndexJ7);

actionOut = [mean(abstractActionJ6(actionIndexJ6,2)), mean(abstractActionJ7(actionIndexJ7,2))];

== matlab function BBC_ensemble_other/Ensemble Control System/highest and average based on pred/averaged action ==
  data: actionJ6 input; actionJ7 input; finalAction output; predications input
function finalAction = fcn(actionJ6, actionJ7, predications)

% average of actions with top 3 highest predicted rewards

allActions = [actionJ6, actionJ7];

selectPred = predications(predications>=0);

if isempty(selectPred)
    actionPred = cat(2, allActions,predications);
    actionPred = sortrows(actionPred,3,'descend');
    finalAction = [mean(actionPred(1:3,1)),mean(actionPred(1:3,2))];
else
    selectAction = allActions(predications>=0,:);
    actionPred = cat(2, selectAction,selectPred);
    actionPred = sortrows(actionPred,3,'descend');
    [num,~] = size(actionPred);
    if num <3
        finalAction = [mean(actionPred(:,1)),mean(actionPred(:,2))];
    else
        finalAction = [mean(actionPred(1:3,1)),mean(actionPred(1:3,2))];
    end

end

== matlab function BBC_ensemble_other/Ensemble Control System/highest and average based on pred/one action ==
  data: actionJ6 input; finalAction output; actionJ7 input; predications input
function finalAction = fcn(actionJ6, actionJ7,predications)

% take the action with highest predicted reward
[~, idx] = max(predications);
finalAction = [actionJ6(idx),actionJ7(idx)];
